simulink model "ballonplate_correctordinates29062016"  (R2016a)
settings: Solver=ode3  StartTime=0.0  StopTime=100  FixedStep=T  RelTol=1e-3
values from neighbouring files (symbols this model uses):
  T = 0.01    [paramters.m]
undefined symbols (not defined in the file or in its folder): initial_position, initial_velocity
libraries: vrlib x10, simulink x5, fuzblock x2
settings Model: Creator=akhan  LastModifiedBy=akhan
settings DataIOCC: LimitDataPoints=on  SaveFormat=Array
settings DebuggingCC: SolverPrmCheckMsg=warning
settings HardwareCC: ProdBitPerPointer=32  ProdLargestAtomicFloat=None  ProdIntDivRoundTo=Undefined  ProdEndianess=Unspecified  ProdWordSize=32  ProdHWDeviceType=32-bit Generic
settings ModelReferenceCC: PropagateSignalLabelsOutOfModel=off
settings ConfigComp: CovModelRefEnable=Off  CovSFcnEnable=off

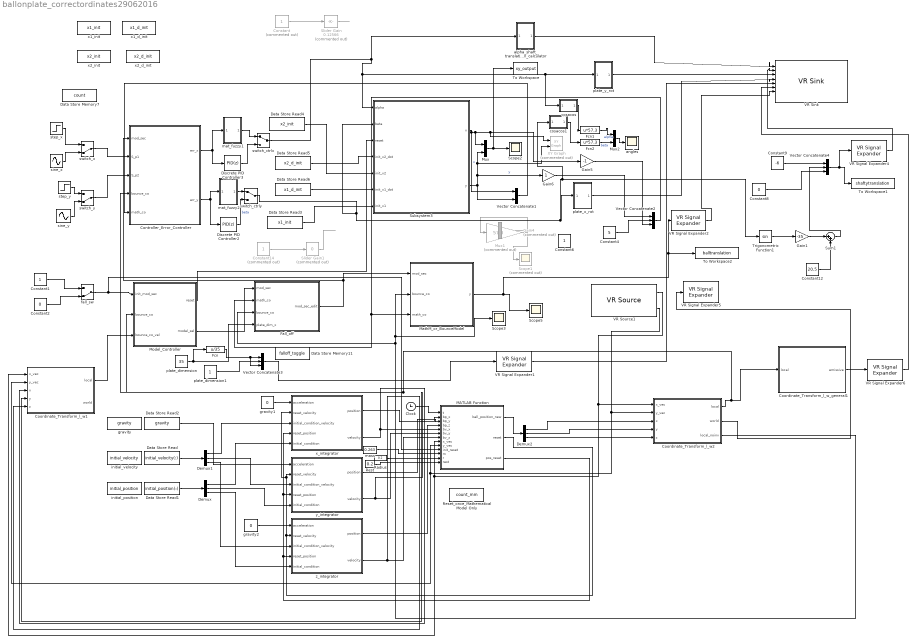
== system ballonplate_correctordinates29062016 ==
  Clock : Clock
  Constant : Constant  Commented=on
  Constant1 : Constant
  Constant12 : Constant  Value=20.5
  Constant14 : Constant  Commented=on
  Constant2 : Constant  Value=0
  Constant4 : Constant  Value=5
  Constant6 : Constant
  Constant8 : Constant  Value=0
  Constant9 : Constant  Value=-6
  Controller_Error_Controller : MATLAB Function  TreatAsAtomicUnit=on
  Coordinate_Transform_l_w1 : MATLAB Function  TreatAsAtomicUnit=on
  Coordinate_Transform_l_w2 : MATLAB Function  TreatAsAtomicUnit=on
  Coordinate_Transform_l_w_general1 : MATLAB Function  TreatAsAtomicUnit=on
  Data Store Memory11 : DataStoreMemory  DataStoreName=falloff_toggle  ShowAdditionalParam=off  OutDataTypeStr=double
  Data Store Memory7 : DataStoreMemory  DataStoreName=count  ShowAdditionalParam=off  OutDataTypeStr=double
  Data Store Read : DataStoreRead  DataStoreName=initial_velocity  DataStoreElements=initial_velocity(:)
  Data Store Read1 : DataStoreRead  DataStoreName=initial_position  DataStoreElements=initial_position(:)
  Data Store Read2 : DataStoreRead  DataStoreName=gravity  DataStoreElements=gravity
  Data Store Read3 : DataStoreRead  DataStoreName=x1_init  DataStoreElements=x1_init
  Data Store Read4 : DataStoreRead  DataStoreName=x2_init  DataStoreElements=x2_init
  Data Store Read5 : DataStoreRead  DataStoreName=x2_d_init  DataStoreElements=x2_d_init
  Data Store Read6 : DataStoreRead  DataStoreName=x1_d_init  DataStoreElements=x1_d_init
  Demux : Demux  Outputs=3
  Demux1 : Demux  Outputs=3
  Demux2 : Demux  Outputs=3
  Discrete PID Controller2 : simulink/Continuous/PID Controller  Controller=PID  TimeDomain=Discrete-time  SampleTime=T  IntegratorMethod=Backward Euler  FilterMethod=Forward Euler  Form=Parallel  UseFilter=on  ControllerParametersSource=internal  P=0.0496279719669994  I=0.00120600765535881  D=0.453206483387622  N=36.9012017074974  InitialConditionSource=internal  InitialConditionForIntegrator=0  InitialConditionForFilter=0  ExternalReset=none  LimitOutput=on  UpperSaturationLimit=1  LowerSaturationLimit=-1  LinearizeAsGain=off  AntiWindupMode=none  Kb=1  TrackingMode=off  Kt=1  PParamMin=[]  PParamMax=[]  IParamMin=[]  IParamMax=[]  DParamMin=[]  DParamMax=[]  NParamMin=[]  NParamMax=[]  KbParamMin=[]  KbParamMax=[]  KtParamMin=[]  KtParamMax=[]  POutMin=[]  POutMax=[]  IOutMin=[]  IOutMax=[]  DOutMin=[]  DOutMax=[]  NOutMin=[]  NOutMax=[]  KbOutMin=[]  KbOutMax=[]  KtOutMin=[]  KtOutMax=[]  IntegratorOutMin=[]  IntegratorOutMax=[]  FilterOutMin=[]  FilterOutMax=[]  SumOutMin=[]  SumOutMax=[]  SumI1OutMin=[]  SumI1OutMax=[]  SumI2OutMin=[]  SumI2OutMax=[]  SumI3OutMin=[]  SumI3OutMax=[]  SumDOutMin=[]  SumDOutMax=[]  SaturationOutMin=[]  SaturationOutMax=[]  IntegratorContinuousStateAttributes=''  IntegratorStateMustResolveToSignalObject=off  IntegratorRTWStateStorageClass=Auto  FilterContinuousStateAttributes=''  FilterStateMustResolveToSignalObject=off  FilterRTWStateStorageClass=Auto  DifferentiatorICPrevScaledInput=0  DifferentiatorOutMin=[]  DifferentiatorOutMax=[]
  Discrete PID Controller3 : simulink/Continuous/PID Controller  Controller=PID  TimeDomain=Discrete-time  SampleTime=T  IntegratorMethod=Backward Euler  FilterMethod=Forward Euler  Form=Parallel  UseFilter=on  ControllerParametersSource=internal  P=0.0496279719669994  I=0.00120600765535881  D=0.453206483387622  N=36.9012017074974  InitialConditionSource=internal  InitialConditionForIntegrator=0  InitialConditionForFilter=0  ExternalReset=none  LimitOutput=on  UpperSaturationLimit=1  LowerSaturationLimit=-1  LinearizeAsGain=off  AntiWindupMode=none  Kb=1  TrackingMode=off  Kt=1  PParamMin=[]  PParamMax=[]  IParamMin=[]  IParamMax=[]  DParamMin=[]  DParamMax=[]  NParamMin=[]  NParamMax=[]  KbParamMin=[]  KbParamMax=[]  KtParamMin=[]  KtParamMax=[]  POutMin=[]  POutMax=[]  IOutMin=[]  IOutMax=[]  DOutMin=[]  DOutMax=[]  NOutMin=[]  NOutMax=[]  KbOutMin=[]  KbOutMax=[]  KtOutMin=[]  KtOutMax=[]  IntegratorOutMin=[]  IntegratorOutMax=[]  FilterOutMin=[]  FilterOutMax=[]  SumOutMin=[]  SumOutMax=[]  SumI1OutMin=[]  SumI1OutMax=[]  SumI2OutMin=[]  SumI2OutMax=[]  SumI3OutMin=[]  SumI3OutMax=[]  SumDOutMin=[]  SumDOutMax=[]  SaturationOutMin=[]  SaturationOutMax=[]  IntegratorContinuousStateAttributes=''  IntegratorStateMustResolveToSignalObject=off  IntegratorRTWStateStorageClass=Auto  FilterContinuousStateAttributes=''  FilterStateMustResolveToSignalObject=off  FilterRTWStateStorageClass=Auto  DifferentiatorICPrevScaledInput=0  DifferentiatorOutMin=[]  DifferentiatorOutMax=[]
  Fall_off : MATLAB Function  TreatAsAtomicUnit=on
  Fcn : Fcn  Expr=u/35
  Fcn1 : Fcn  Expr=u*57.3
  Fcn2 : Fcn  Expr=u*57.3
  Gain1 : Gain  Gain=-35
  Gain4 : Gain  Commented=on  Gain=57.3  SampleTime=T
  Gain5 : Gain  Gain=-1
  Gain6 : Gain
  MATLAB Function : MATLAB Function  TreatAsAtomicUnit=on
  MathM_or_BounceModel : MATLAB Function  TreatAsAtomicUnit=on
  Model_Controller : MATLAB Function  TreatAsAtomicUnit=on
  Mux : Mux  Inputs=2
  Mux1 : Mux  Commented=on  Inputs=2
  Mux2 : Mux  Inputs=2
  Radius : Constant  Value=0.2
  Reset_once_Mathematical Model Only : DataStoreMemory  DataStoreName=count_mm  ShowAdditionalParam=off  OutDataTypeStr=double
  Rest : Constant  Value=0.2
  Scope1 : Scope  Commented=on
  Scope2 : Scope
  Scope3 : Scope
  Scope5 : Scope
  Slider Gain : simulink/Math Operations/Slider Gain  Commented=on  low=-1.5708  gain=0.12566  high=1.5708
  Slider Gain1 : simulink/Math Operations/Slider Gain  Commented=on  low=-1.5708  gain=0  high=1.57
  Subsystem3 : Subsystem  mask{m=0.263, r=0.2}
      mask prompts: m "Mass"; r "Radius"
      mask Display:
      | image('bp.jpg')
      | port_label('input',1,'alpha')
      | port_label('input',2,'beta')
      | port_label('input',3,'reset')
      | port_label('input',4,'x2_dot_init')
      | port_label('input',5,'x2_init')
      | port_label('input',6,'x1_dot_init')
      | port_label('input',7,'x1_init')
      | port_label('output',1,'x')
      | port_label('output',2,'y')
  Sum1 : Sum  Inputs=|++
  To Workspace : ToWorkspace  VariableName=xy_output  SaveFormat=Timeseries  SampleTime=T
  To Workspace1 : ToWorkspace  VariableName=shaftytranslation  SaveFormat=Timeseries  SampleTime=T
  To Workspace2 : ToWorkspace  VariableName=balltranslation  SaveFormat=Timeseries  SampleTime=T
  Trigonometric Function1 : Trigonometry
  VR Signal Expander{1,4..6} (4 alike) : vrlib/VR Signal Expander  outwidth=3  outidx=[1 2 3]
  VR Signal Expander2 : vrlib/VR Signal Expander  outwidth=3  outidx=[3 2 1]
  VR Sink : vrlib/VR Sink  InstantiateOnLoad=on  SampleTime=-1  ViewEnable=on  RemoteChange=off  RemoteView=off  FieldsWritten=shaft_x.translation.3.1.1.double#shaft_y.translation.3.1.1.double#plate_test_y.rotation.4.1.1.double#plate_test_x.rotation.4.1.1.double#plate_trans.scale.3.1.1.double#plate_mat.emissiveColor.3.1.1.double#ball_trans.translation.3.1.1.double#world_ball.translation.3.1.1.double  WorldFileName=bandplate_move_correctordinates.wrl  AutoView=off  VideoDimensions=[]  AllowVariableSize=off
  VR Source1 : vrlib/VR Source  InstantiateOnLoad=on  SampleTime=-1  ViewEnable=on  RemoteChange=off  RemoteView=off  FieldsRead=reference_x.translation_abs.1.3.1.double#reference_y.translation_abs.1.3.1.double  WorldFileName=bandplate_move_correctordinates.wrl  AutoView=off  VideoDimensions=[]  AllowVariableSize=off
  Vector Concatenate1 : Concatenate
  Vector Concatenate2 : Concatenate  NumInputs=3
  Vector Concatenate3 : Concatenate  NumInputs=3
  Vector Concatenate4 : Concatenate  NumInputs=3
  XY Graph : simulink/Sinks/XY Graph  Commented=on  xmin=-35  xmax=35  ymin=-35  ymax=35  st=-1
  alpha_shaft_translation_calculator : Subsystem
  angles : Scope
  cosacos : Subsystem
  cosacos1 : Subsystem
  fall_sw : ManualSwitch  CurrentSetting=0
  gravity : DataStoreMemory  DataStoreName=gravity  InitialValue=-4  ShowAdditionalParam=off  OutDataTypeStr=double
  gravity1 : Constant  Value=0
  gravity2 : Constant  Value=0
  initial_position : DataStoreMemory  DataStoreName=initial_position  InitialValue=[5;25;3]  ShowAdditionalParam=off  OutDataTypeStr=double
  initial_velocity : DataStoreMemory  DataStoreName=initial_velocity  InitialValue=[0;5;0]  ShowAdditionalParam=off  OutDataTypeStr=double
  mass : Constant  Value=0.263
  mat_fuzzy1 : Subsystem
  mat_fuzzy2 : Subsystem
  plate_dimension : Constant  Value=35
  plate_dimension1 : Constant
  plate_x_rot : Subsystem
  plate_y_rot : Subsystem
  sine_x : Sin  Amplitude=5  Frequency=0.1  SampleTime=0
  sine_y : Sin  Amplitude=5  Frequency=0.1  Phase=-pi/2  SampleTime=0
  step_x : Step  Time=0  After=5  SampleTime=0
  step_y : Step  Time=0  After=5  SampleTime=0
  switch_ctrlx : ManualSwitch
  switch_ctrly : ManualSwitch
  switch_x : ManualSwitch  CurrentSetting=0
  switch_y : ManualSwitch  CurrentSetting=0
  x1_d_init : DataStoreMemory  DataStoreName=x1_d_init  ShowAdditionalParam=off  OutDataTypeStr=double
  x1_init : DataStoreMemory  DataStoreName=x1_init  ShowAdditionalParam=off  OutDataTypeStr=double
  x2_d_init : DataStoreMemory  DataStoreName=x2_d_init  ShowAdditionalParam=off  OutDataTypeStr=double
  x2_init : DataStoreMemory  DataStoreName=x2_init  ShowAdditionalParam=off  OutDataTypeStr=double
  x_integrator : Subsystem
  y_integrator : Subsystem
  z_integrator : Subsystem
  wires:
  Subsystem3/1(x) -> Vector Concatenate1/1, XY Graph/1, Gain5/1, Mux/1  "x"
  Subsystem3/2(y) -> XY Graph/2, Mux/2, Gain6/1, Vector Concatenate1/2  "y"
  Mux1/1 -> Gain4/1
  Gain4/1 -> Scope1/1
  Constant4/1 -> Vector Concatenate2/2
  Vector Concatenate2/1 -> Fall_off/2(math_co), MathM_or_BounceModel/3(math_co)
  Vector Concatenate4/1 -> To Workspace1/1, VR Signal Expander4/1
  Constant9/1 -> Vector Concatenate4/1
  Constant8/1 -> Vector Concatenate4/3
  Trigonometric Function1/1 -> Gain1/1
  Gain1/1 -> Sum1/1
  Constant12/1 -> Sum1/2
  Sum1/1 -> Vector Concatenate4/2
  Gain5/1 -> Vector Concatenate2/3
  Gain6/1 -> Vector Concatenate2/1
  Constant/1 -> Slider Gain/1
  Constant14/1 -> Slider Gain1/1
  Slider Gain/1 -> ?
  switch_ctrlx/1 -> Subsystem3/1(alpha), cosacos/1(In1), plate_y_rot/1(In1), alpha_shaft_translation_calculator/1(In1)
  Slider Gain1/1 -> ?
  switch_ctrly/1 -> cosacos1/1(In1), Trigonometric Function1/1, plate_x_rot/1(In1), Subsystem3/2(beta)
  VR Source1/1 -> Coordinate_Transform_l_w2/1(x_vec), MATLAB Function/8(x_vec), Coordinate_Transform_l_w1/1(x_vec)
  VR Source1/2 -> Coordinate_Transform_l_w2/2(y_vec), MATLAB Function/9(y_vec), Coordinate_Transform_l_w1/2(y_vec)
  Coordinate_Transform_l_w2/2(world) -> VR Signal Expander5/1
  Coordinate_Transform_l_w2/1(local) -> Controller_Error_Controller/4(bounce_co), Model_Controller/2(bounce_co), Coordinate_Transform_l_w_general1/1(local)
  Coordinate_Transform_l_w_general1/1(emissive) -> VR Signal Expander6/1
  Data Store Read2/1 -> y_integrator/1(acceleration)
  x_integrator/1(position) -> MATLAB Function/2(bp_x)
  y_integrator/1(position) -> MATLAB Function/3(bp_y)
  z_integrator/1(position) -> MATLAB Function/4(bp_z)
  x_integrator/2(velocity) -> Coordinate_Transform_l_w1/3(x), MATLAB Function/5(bv_x)
  y_integrator/2(velocity) -> Coordinate_Transform_l_w1/4(y), MATLAB Function/6(bv_y)
  z_integrator/2(velocity) -> Coordinate_Transform_l_w1/5(z), MATLAB Function/7(bv_z)
  Demux/1 -> x_integrator/5(initial_condition)
  Demux/2 -> y_integrator/5(initial_condition)
  Demux/3 -> z_integrator/5(initial_condition)
  Demux1/1 -> x_integrator/3(initial_condition_velocity)
  Demux1/2 -> y_integrator/3(initial_condition_velocity)
  Demux1/3 -> z_integrator/3(initial_condition_velocity)
  gravity1/1 -> x_integrator/1(acceleration)
  gravity2/1 -> z_integrator/1(acceleration)
  MATLAB Function/1(ball_position_new) -> Demux2/1
  Demux2/1 -> Coordinate_Transform_l_w2/3(x)
  Demux2/2 -> Coordinate_Transform_l_w2/4(y)
  Demux2/3 -> Coordinate_Transform_l_w2/5(z)
  MATLAB Function/2(reset) -> z_integrator/2(reset_velocity), x_integrator/2(reset_velocity), y_integrator/2(reset_velocity)
  Data Store Read/1 -> Demux1/1
  Data Store Read1/1 -> Demux/1
  MATLAB Function/3(pos_reset) -> x_integrator/4(reset_position), y_integrator/4(reset_position), z_integrator/4(reset_position)
  Clock/1 -> MATLAB Function/1(t)
  Mux/1 -> To Workspace/1, Scope2/1
  Data Store Read5/1 -> Subsystem3/4(init_x2_dot)
  Data Store Read6/1 -> Subsystem3/6(init_x1_dot)
  Data Store Read4/1 -> Subsystem3/5(init_x2)
  Data Store Read3/1 -> Subsystem3/7(init_x1)
  Model_Controller/1(reset) -> Subsystem3/3(reset)
  Coordinate_Transform_l_w2/3(local_noinv) -> Fall_off/3(bounce_co), MathM_or_BounceModel/2(bounce_co), Scope3/1
  fall_sw/1 -> MATLAB Function/10(init_reset), Model_Controller/1(init_mod_sec)
  Constant1/1 -> fall_sw/1
  Constant2/1 -> fall_sw/2
  Vector Concatenate1/1 -> Controller_Error_Controller/5(math_co)
  Coordinate_Transform_l_w1/1(local) -> Model_Controller/3(bounce_co_vel)
  Model_Controller/2(model_sel) -> Fall_off/1(mod_sec)
  Fall_off/1(mod_sec_edit) -> Controller_Error_Controller/1(mod_sec), MathM_or_BounceModel/1(mod_sec)
  MathM_or_BounceModel/1(y) -> To Workspace2/1, VR Signal Expander2/1, Scope5/1
  step_y/1 -> switch_y/1
  sine_y/1 -> switch_y/2
  switch_y/1 -> Controller_Error_Controller/3(S_p2)
  switch_x/1 -> Controller_Error_Controller/2(S_p1)
  sine_x/1 -> switch_x/2
  plate_dimension/1 -> Fcn/1, Fall_off/4(plate_dim_x)
  alpha_shaft_translation_calculator/1(Out1) -> VR Sink/1
  VR Signal Expander4/1 -> VR Sink/2
  plate_y_rot/1(Out1) -> VR Sink/3
  plate_x_rot/1(Out1) -> VR Sink/4
  VR Signal Expander6/1 -> VR Sink/6
  VR Signal Expander2/1 -> VR Sink/7
  Fcn/1 -> Vector Concatenate3/3, Vector Concatenate3/1
  plate_dimension1/1 -> Vector Concatenate3/2
  Vector Concatenate3/1 -> VR Signal Expander1/1
  VR Signal Expander1/1 -> VR Sink/5
  Rest/1 -> MATLAB Function/13(rest)
  mass/1 -> MATLAB Function/11(m)
  Radius/1 -> MATLAB Function/12(r)
  Fcn1/1 -> Mux2/1  "alpha"
  Fcn2/1 -> Mux2/2  "beta"
  Mux2/1 -> angles/1
  cosacos/1(Out1) -> Fcn1/1
  cosacos1/1(Out1) -> Fcn2/1
  Controller_Error_Controller/2(err_y) -> Discrete PID Controller2/1, mat_fuzzy2/1(In1)
  step_x/1 -> switch_x/1
  mat_fuzzy1/1(Out1) -> switch_ctrlx/1
  Discrete PID Controller3/1 -> switch_ctrlx/2
  Controller_Error_Controller/1(err_x) -> Discrete PID Controller3/1, mat_fuzzy1/1(In1)
  mat_fuzzy2/1(Out1) -> switch_ctrly/1
  Discrete PID Controller2/1 -> switch_ctrly/2  "beta"

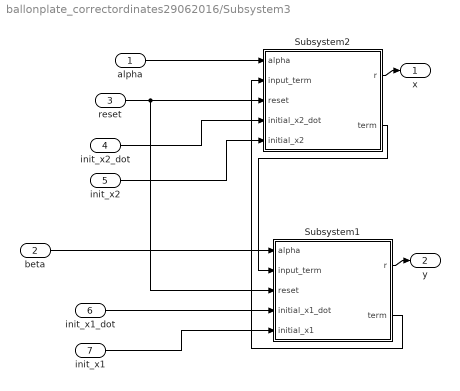
== system ballonplate_correctordinates29062016/Subsystem3 ==
  alpha : Inport
  beta : Inport  Port=2
  reset : Inport  Port=3
  init_x2_dot : Inport  Port=4
  init_x2 : Inport  Port=5
  init_x1_dot : Inport  Port=6
  init_x1 : Inport  Port=7
  Subsystem1 : Subsystem
  Subsystem2 : Subsystem
  x : Outport
  y : Outport  Port=2
  wires:
  Subsystem1/2(term) -> Subsystem2/2(input_term)
  beta/1 -> Subsystem1/1(alpha)
  alpha/1 -> Subsystem2/1(alpha)
  Subsystem1/1(r) -> y/1
  Subsystem2/1(r) -> x/1
  Subsystem2/2(term) -> Subsystem1/2(input_term)
  reset/1 -> Subsystem1/3(reset), Subsystem2/3(reset)
  init_x2_dot/1 -> Subsystem2/4(initial_x2_dot)
  init_x2/1 -> Subsystem2/5(initial_x2)
  init_x1_dot/1 -> Subsystem1/4(initial_x1_dot)
  init_x1/1 -> Subsystem1/5(initial_x1)

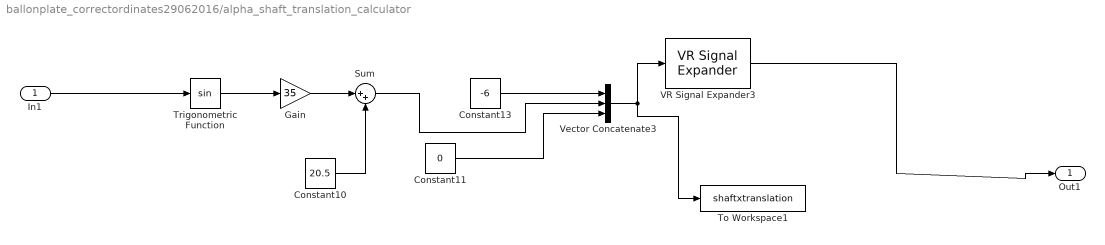
== system ballonplate_correctordinates29062016/alpha_shaft_translation_calculator ==
  In1 : Inport
  Constant10 : Constant  Value=20.5
  Constant11 : Constant  Value=0
  Constant13 : Constant  Value=-6
  Gain : Gain  Gain=35
  Sum : Sum  Inputs=|++
  To Workspace1 : ToWorkspace  VariableName=shaftxtranslation  SaveFormat=Timeseries  SampleTime=T
  Trigonometric Function : Trigonometry
  VR Signal Expander3 : vrlib/VR Signal Expander  outwidth=3  outidx=[1 2 3]
  Vector Concatenate3 : Concatenate  NumInputs=3
  Out1 : Outport
  wires:
  Constant11/1 -> Vector Concatenate3/3
  Vector Concatenate3/1 -> VR Signal Expander3/1, To Workspace1/1
  Constant13/1 -> Vector Concatenate3/1
  Gain/1 -> Sum/1
  Constant10/1 -> Sum/2
  Trigonometric Function/1 -> Gain/1
  Sum/1 -> Vector Concatenate3/2
  VR Signal Expander3/1 -> Out1/1
  In1/1 -> Trigonometric Function/1

== system ballonplate_correctordinates29062016/cosacos ==
  In1 : Inport
  Trigonometric Function3 : Trigonometry  Operator=acos
  Trigonometric Function4 : Trigonometry  Operator=cos
  Out1 : Outport
  wires:
  In1/1 -> Trigonometric Function4/1
  Trigonometric Function3/1 -> Out1/1
  Trigonometric Function4/1 -> Trigonometric Function3/1

== system ballonplate_correctordinates29062016/cosacos1 ==
  In1 : Inport
  Trigonometric Function3 : Trigonometry  Operator=acos
  Trigonometric Function4 : Trigonometry  Operator=cos
  Out1 : Outport
  wires:
  In1/1 -> Trigonometric Function4/1
  Trigonometric Function3/1 -> Out1/1
  Trigonometric Function4/1 -> Trigonometric Function3/1

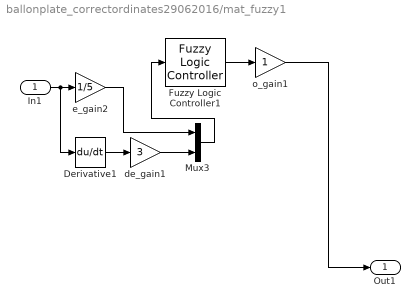
== system ballonplate_correctordinates29062016/mat_fuzzy1 ==
  In1 : Inport
  Derivative1 : Derivative
  Fuzzy Logic Controller1 : fuzblock/Fuzzy Logic  Controller  fis='ball_plate_normalized.fis'
  Mux3 : Mux  Inputs=2
  de_gain1 : Gain  Gain=3
  e_gain2 : Gain  Gain=1/5
  o_gain1 : Gain
  Out1 : Outport
  wires:
  e_gain2/1 -> Mux3/1
  Mux3/1 -> Fuzzy Logic Controller1/1
  Fuzzy Logic Controller1/1 -> o_gain1/1
  de_gain1/1 -> Mux3/2
  Derivative1/1 -> de_gain1/1
  In1/1 -> Derivative1/1, e_gain2/1
  o_gain1/1 -> Out1/1

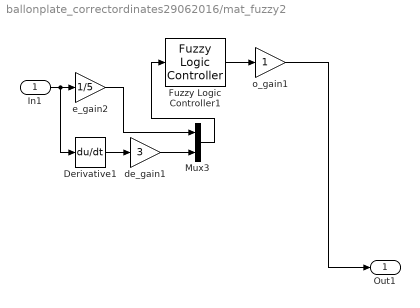
== system ballonplate_correctordinates29062016/mat_fuzzy2 ==
  In1 : Inport
  Derivative1 : Derivative
  Fuzzy Logic Controller1 : fuzblock/Fuzzy Logic  Controller  fis='ball_plate_normalized.fis'
  Mux3 : Mux  Inputs=2
  de_gain1 : Gain  Gain=3
  e_gain2 : Gain  Gain=1/5
  o_gain1 : Gain
  Out1 : Outport
  wires:
  e_gain2/1 -> Mux3/1
  Mux3/1 -> Fuzzy Logic Controller1/1
  Fuzzy Logic Controller1/1 -> o_gain1/1
  de_gain1/1 -> Mux3/2
  Derivative1/1 -> de_gain1/1
  In1/1 -> Derivative1/1, e_gain2/1
  o_gain1/1 -> Out1/1

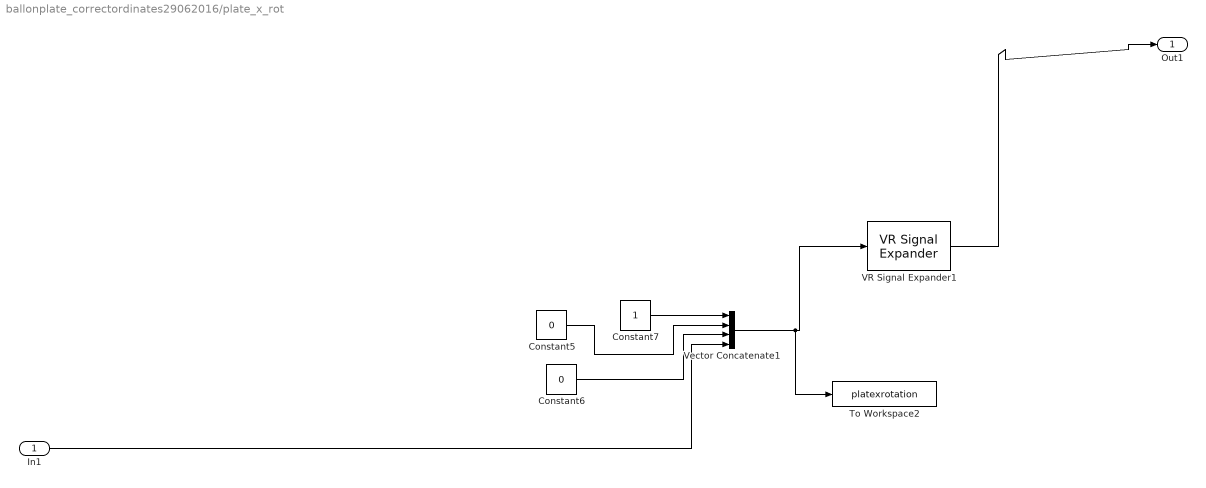
== system ballonplate_correctordinates29062016/plate_x_rot ==
  In1 : Inport
  Constant5 : Constant  Value=0
  Constant6 : Constant  Value=0
  Constant7 : Constant
  To Workspace2 : ToWorkspace  VariableName=platexrotation  SaveFormat=Timeseries  SampleTime=T
  VR Signal Expander1 : vrlib/VR Signal Expander  outwidth=4  outidx=[1 2 3 4]
  Vector Concatenate1 : Concatenate  NumInputs=4
  Out1 : Outport
  wires:
  Constant6/1 -> Vector Concatenate1/3
  Constant5/1 -> Vector Concatenate1/2
  Vector Concatenate1/1 -> To Workspace2/1, VR Signal Expander1/1
  Constant7/1 -> Vector Concatenate1/1
  VR Signal Expander1/1 -> Out1/1
  In1/1 -> Vector Concatenate1/4

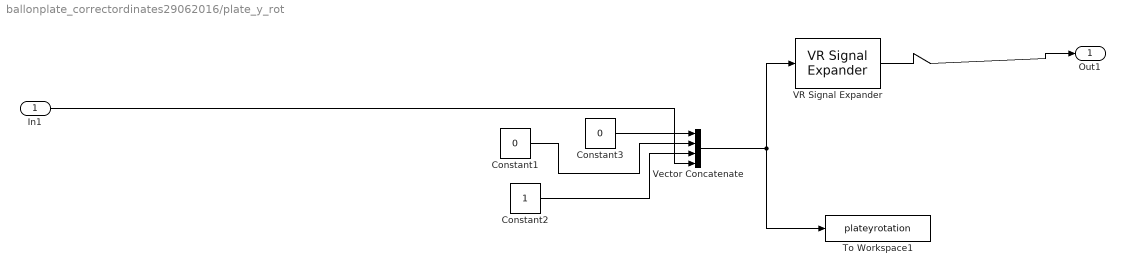
== system ballonplate_correctordinates29062016/plate_y_rot ==
  In1 : Inport
  Constant1 : Constant  Value=0
  Constant2 : Constant
  Constant3 : Constant  Value=0
  To Workspace1 : ToWorkspace  VariableName=plateyrotation  SaveFormat=Timeseries  SampleTime=-1
  VR Signal Expander : vrlib/VR Signal Expander  outwidth=4  outidx=[1 2 3 4]
  Vector Concatenate : Concatenate  NumInputs=4
  Out1 : Outport
  wires:
  Vector Concatenate/1 -> To Workspace1/1, VR Signal Expander/1
  Constant2/1 -> Vector Concatenate/3
  Constant1/1 -> Vector Concatenate/2
  Constant3/1 -> Vector Concatenate/1
  VR Signal Expander/1 -> Out1/1
  In1/1 -> Vector Concatenate/4

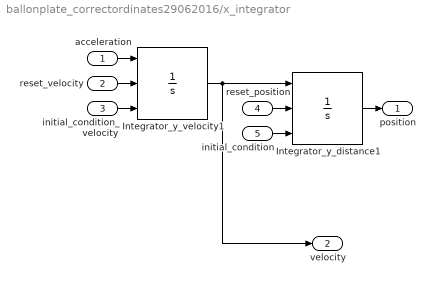
== system ballonplate_correctordinates29062016/x_integrator ==
  acceleration : Inport
  reset_velocity : Inport  Port=2
  initial_condition_velocity : Inport  Port=3
  reset_position : Inport  Port=4
  initial_condition : Inport  Port=5
  Integrator_y_distance1 : Integrator  ExternalReset=rising  InitialConditionSource=external
  Integrator_y_velocity1 : Integrator  ExternalReset=rising  InitialConditionSource=external
  position : Outport
  velocity : Outport  Port=2
  wires:
  Integrator_y_velocity1/1 -> velocity/1, Integrator_y_distance1/1
  reset_position/1 -> Integrator_y_distance1/2
  Integrator_y_distance1/1 -> position/1
  initial_condition_velocity/1 -> Integrator_y_velocity1/3
  initial_condition/1 -> Integrator_y_distance1/3
  reset_velocity/1 -> Integrator_y_velocity1/2
  acceleration/1 -> Integrator_y_velocity1/1

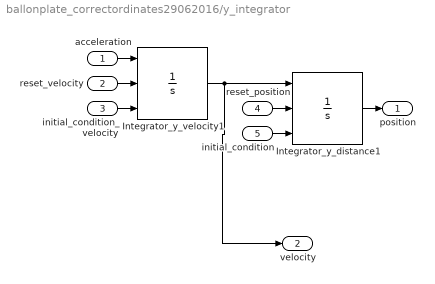
== system ballonplate_correctordinates29062016/y_integrator ==
  acceleration : Inport
  reset_velocity : Inport  Port=2
  initial_condition_velocity : Inport  Port=3
  reset_position : Inport  Port=4
  initial_condition : Inport  Port=5
  Integrator_y_distance1 : Integrator  ExternalReset=rising  InitialConditionSource=external
  Integrator_y_velocity1 : Integrator  ExternalReset=rising  InitialConditionSource=external
  position : Outport
  velocity : Outport  Port=2
  wires:
  Integrator_y_velocity1/1 -> velocity/1, Integrator_y_distance1/1
  reset_position/1 -> Integrator_y_distance1/2
  Integrator_y_distance1/1 -> position/1
  initial_condition_velocity/1 -> Integrator_y_velocity1/3
  initial_condition/1 -> Integrator_y_distance1/3
  reset_velocity/1 -> Integrator_y_velocity1/2
  acceleration/1 -> Integrator_y_velocity1/1

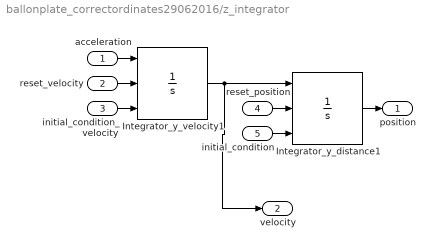
== system ballonplate_correctordinates29062016/z_integrator ==
  acceleration : Inport
  reset_velocity : Inport  Port=2
  initial_condition_velocity : Inport  Port=3
  reset_position : Inport  Port=4
  initial_condition : Inport  Port=5
  Integrator_y_distance1 : Integrator  ExternalReset=rising  InitialConditionSource=external
  Integrator_y_velocity1 : Integrator  ExternalReset=rising  InitialConditionSource=external
  position : Outport
  velocity : Outport  Port=2
  wires:
  Integrator_y_velocity1/1 -> velocity/1, Integrator_y_distance1/1
  reset_position/1 -> Integrator_y_distance1/2
  Integrator_y_distance1/1 -> position/1
  initial_condition_velocity/1 -> Integrator_y_velocity1/3
  initial_condition/1 -> Integrator_y_distance1/3
  reset_velocity/1 -> Integrator_y_velocity1/2
  acceleration/1 -> Integrator_y_velocity1/1

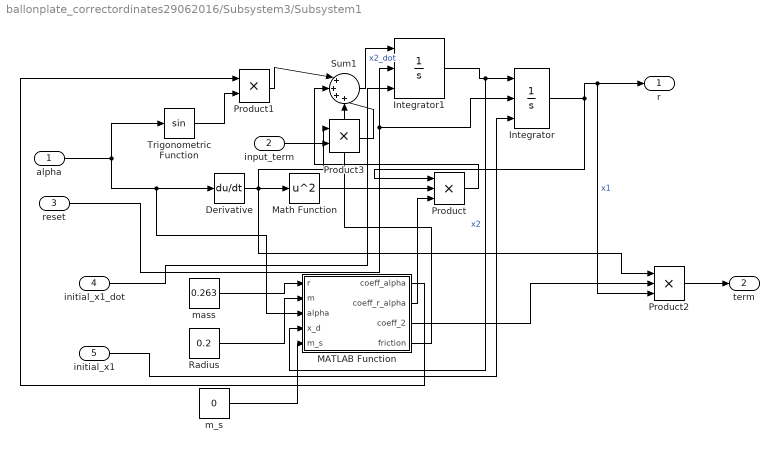
== system ballonplate_correctordinates29062016/Subsystem3/Subsystem1 ==
  alpha : Inport
  input_term : Inport  Port=2
  reset : Inport  Port=3
  initial_x1_dot : Inport  Port=4
  initial_x1 : Inport  Port=5
  Derivative : Derivative
  Integrator : Integrator  ExternalReset=rising  InitialConditionSource=external  InitialCondition=0.004427
  Integrator1 : Integrator  ExternalReset=rising  InitialConditionSource=external
  MATLAB Function : MATLAB Function  TreatAsAtomicUnit=on
  Math Function : Math  Operator=square  SaturateOnIntegerOverflow=on
  Product : Product  Inputs=3
  Product1 : Product
  Product2 : Product  Inputs=3
  Product3 : Product
  Radius : Constant  Value=0.2
  Sum1 : Sum  Inputs=|++++
  Trigonometric Function : Trigonometry
  m_s : Constant  Value=0
  mass : Constant  Value=0.263
  r : Outport
  term : Outport  Port=2
  wires:
  Product1/1 -> Sum1/1
  Derivative/1 -> Product2/1, Product3/1, Math Function/1
  Sum1/1 -> Integrator1/1  "x2_dot"
  Integrator/1 -> Product2/3, r/1, Product/1  "x1"
  Product/1 -> Sum1/2
  Integrator1/1 -> MATLAB Function/4(x_d), Integrator/1  "x2"
  Trigonometric Function/1 -> Product1/2
  alpha/1 -> MATLAB Function/3(alpha), Derivative/1, Trigonometric Function/1
  Math Function/1 -> Product/2
  mass/1 -> MATLAB Function/1(r)
  Radius/1 -> MATLAB Function/2(m)
  MATLAB Function/1(coeff_alpha) -> Product1/1
  MATLAB Function/2(coeff_r_alpha) -> Product/3
  MATLAB Function/3(coeff_2) -> Product2/2
  Product2/1 -> term/1
  input_term/1 -> Product3/2
  Product3/1 -> Sum1/3
  reset/1 -> Integrator/2, Integrator1/2
  initial_x1_dot/1 -> Integrator1/3
  initial_x1/1 -> Integrator/3
  MATLAB Function/4(friction) -> Sum1/4
  m_s/1 -> MATLAB Function/5(m_s)

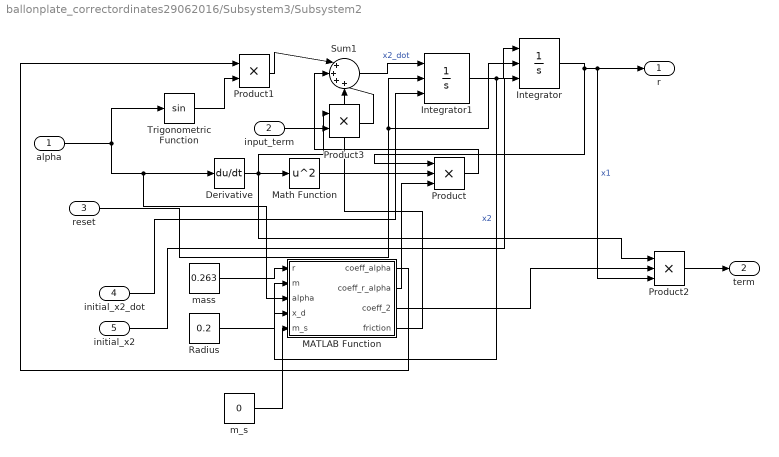
== system ballonplate_correctordinates29062016/Subsystem3/Subsystem2 ==
  alpha : Inport
  input_term : Inport  Port=2
  reset : Inport  Port=3
  initial_x2_dot : Inport  Port=4
  initial_x2 : Inport  Port=5
  Derivative : Derivative
  Integrator : Integrator  ExternalReset=rising  InitialConditionSource=external  InitialCondition=0.004427
  Integrator1 : Integrator  ExternalReset=rising  InitialConditionSource=external
  MATLAB Function : MATLAB Function  TreatAsAtomicUnit=on
  Math Function : Math  Operator=square  SaturateOnIntegerOverflow=on
  Product : Product  Inputs=3
  Product1 : Product
  Product2 : Product  Inputs=3
  Product3 : Product
  Radius : Constant  Value=0.2
  Sum1 : Sum  Inputs=|++++
  Trigonometric Function : Trigonometry
  m_s : Constant  Value=0
  mass : Constant  Value=0.263
  r : Outport
  term : Outport  Port=2
  wires:
  Product1/1 -> Sum1/1
  Derivative/1 -> Product2/1, Product3/1, Math Function/1
  Sum1/1 -> Integrator1/1  "x2_dot"
  Integrator/1 -> Product/1, Product2/3, r/1  "x1"
  Product/1 -> Sum1/2
  Integrator1/1 -> MATLAB Function/4(x_d), Integrator/1  "x2"
  Trigonometric Function/1 -> Product1/2
  alpha/1 -> MATLAB Function/3(alpha), Derivative/1, Trigonometric Function/1
  Math Function/1 -> Product/2
  mass/1 -> MATLAB Function/1(r)
  Radius/1 -> MATLAB Function/2(m)
  MATLAB Function/1(coeff_alpha) -> Product1/1
  MATLAB Function/2(coeff_r_alpha) -> Product/3
  MATLAB Function/3(coeff_2) -> Product2/2
  Product2/1 -> term/1
  input_term/1 -> Product3/2
  Product3/1 -> Sum1/3
  reset/1 -> Integrator/2, Integrator1/2
  initial_x2_dot/1 -> Integrator1/3
  initial_x2/1 -> Integrator/3
  MATLAB Function/4(friction) -> Sum1/4
  m_s/1 -> MATLAB Function/5(m_s)

== matlab function ballonplate_correctordinates29062016/Subsystem3/Subsystem1/MATLAB Function ==
  data: r input; coeff_alpha output; m input; coeff_r_alpha output; coeff_2 output; alpha input; x_d input; friction output; m_s input
function [coeff_alpha, coeff_r_alpha,coeff_2,friction] = fcn(r,m,alpha,x_d,m_s)
%#codeg
J=2*m*r*r/5;
coeff_r_alpha=m/((J/r*r)+m);
coeff_alpha=   -m*(-9.8)/((J/r*r)+m);
coeff_2=m/((J/r*r)+m);


m_s = 0;
friction = -m_s*m*9.8*cos(alpha)*sign(x_d);
friction = friction/((J/r*r)+m);

== matlab function ballonplate_correctordinates29062016/Subsystem3/Subsystem2/MATLAB Function ==
  data: r input; coeff_alpha output; m input; coeff_r_alpha output; coeff_2 output; alpha input; friction output; x_d input; m_s input
function [coeff_alpha, coeff_r_alpha,coeff_2,friction] = fcn(r,m,alpha,x_d,m_s)
%#codeg
J=2*m*r*r/5;
coeff_r_alpha=m/((J/r*r)+m);
coeff_alpha=   -m*(-9.8)/((J/r*r)+m);
coeff_2=m/((J/r*r)+m);


%coefficient of friction

friction = -m_s*m*9.8*cos(alpha)*sign(x_d);
friction = friction/((J/r*r)+m);

== matlab function ballonplate_correctordinates29062016/MathM_or_BounceModel ==
  data: mod_sec input; y output size=3; gravity data_store_memory; bounce_co input size=3; math_co input size=3
function y = fcn(mod_sec,bounce_co,math_co)
%mod_sec if 0 output is bounce_co
%if anything else math_co
%this requires bounce_co and math_co for vrml model, note doesn't require
%the negative
if mod_sec == 1
    y = bounce_co;
elseif mod_sec == 0
    y = math_co;
else
    y = [2000 2000 2000]';
end

== matlab function ballonplate_correctordinates29062016/Controller_Error_Controller ==
  data: mod_sec input; S_p1 input; S_p2 input; err_x output; gravity data_store_memory; bounce_co input; math_co input size=2; err_y output
function [err_x,err_y] = fcn(mod_sec,S_p1,S_p2,bounce_co,math_co)
%this function requires the bounce_co and math_co for the mathematical
%model coordinates
threshold_for_touch = 3;
if mod_sec == 3
err_x = 0;
err_y = 0;
else
    if mod_sec == 0
        err_x = S_p1 - math_co(1);
        err_y = S_p2 - math_co(2);
    %threshold for touch
    elseif bounce_co(3)<= threshold_for_touch
        err_x = S_p1 - bounce_co(1);
        err_y = S_p2 - bounce_co(2);
    else err_x = 0;
         err_y = 0;
    end
end

== matlab function ballonplate_correctordinates29062016/Model_Controller ==
  data: init_mod_sec input; reset output; gravity data_store_memory; bounce_co input; bounce_co_vel input; model_sel output; x1_init data_store_memory; x1_d_init data_store_memory; x2_init data_store_memory; x2_d_init data_store_memory; initial_velocity data_store_memory; initial_position data_store_memory; count data_store_memory
function [reset,model_sel] = fcn(init_mod_sec,bounce_co,bounce_co_vel)
%mod_sec if 0 output is math_co
%if anything else math_co
%this requires the bounce_co in mathematical model coordinates
%probably need a count variable to stop resetting x1_init
global gravity;
global x1_init;
global x1_d_init;
global x2_init;
global x2_d_init;
global initial_velocity;
global initial_position;
global count;



    if init_mod_sec == 0
        gravity = 0;
        model_sel = 0;
        reset = 0;
        initial_position = [0;15;0];
        initial_velocity = [0;0;0];
    else 
        if gravity == 0
            if count <5
                reset = 1;
                x1_init = bounce_co(1);
                x2_init = bounce_co(2);
                x1_d_init = bounce_co_vel(1);
                x2_d_init = bounce_co_vel(2);
                count = count+1;
            else reset =1;
            end
        model_sel = 0;
        
        else reset = 0;
            model_sel = 1;
        end
    end

== matlab function ballonplate_correctordinates29062016/Coordinate_Transform_l_w2 ==
  data: x_vec input; y_vec input; x input; y input; local output; z input; world output; local_noinv output size=[1 3]
function [local,world,local_noinv] = fcn(x_vec,y_vec,x,y,z)
%y_p is y prime which is vector of y coordinate axis after rotation beta
%about the x axis
%x_p is rotation alpha about arbitary axis y_p
%This transformation gives the coordinates in the mathematical model
%coordinates
%x_vec -1 0 0
%y_vec 0 0 1
%z_vec 0 1 0
% This gives local where x is -x therefore x is correct and z 
%just need to swap x and z
world = [x;y;z];
z_vec=cross(x_vec,y_vec);
local=[x_vec,y_vec,z_vec]\[x;y;z];

%this gives local coordinates in vrml frame
local_noinv = [-local(1),local(3),local(2)];

%this gives local coordinates in ball and plate frame
temp = local(1);
local(1) = local(2);
local(2) = temp;

== matlab function ballonplate_correctordinates29062016/Coordinate_Transform_l_w_general1 ==
  data: local input; emissive output
function emissive = fcn(local)

if local(3)<5&(abs(local(2)))<35&(abs(local(3)))<35
    emissive = [0.8 0 0.2];
else emissive = [0 0 0.8];
end

== matlab function ballonplate_correctordinates29062016/MATLAB Function ==
  data: t input; bp_x input; ball_position_new output; bp_y input; bp_z input; bv_x input; bv_y input; bv_z input; reset output; initial_velocity data_store_memory; initial_position data_store_memory; gravity data_store_memory; x_vec input; y_vec input; pos_reset output; count_mm data_store_memory; init_reset input; m input; r input; rest input
function [ball_position_new,reset,pos_reset] = fcn(t,bp_x,bp_y,bp_z,bv_x,bv_y,bv_z,x_vec,y_vec,init_reset,m,r,rest)
%#codegen
global initial_velocity;
global initial_position;
global gravity;
global count_mm;

[local_pos,~]=coordinate_transform(x_vec,y_vec,bp_x,bp_y,bp_z);
ball_position=local_pos;
[local_vel,~]=coordinate_transform(x_vec,y_vec,bv_x,bv_y,bv_z);
ball_velocity=local_vel;
ball_position_new = [bp_x;bp_y;bp_z];
if (ball_position(3)<=3)&&t>0&&gravity~=0&&init_reset~=0
  reset=1;
 pos_reset=0;
% m = 0.263;
% r = 2;
J_sphere =0.4* m*r*r*eye(3);
J_sphere_inv = 2.5*eye(3)/(m*r*r);
% rest = 0.2;
ball_momentum = m*ball_velocity;
%This can change to reflect the plate
m_ground_inv = 0;
J_ground_inv = 0;
N = [0 0 1]';
%ball_position is ball centre which is all centre of gravity
contact_Point = [ball_position(1),ball_position(2),ball_position(3)-r]';
r_ball = contact_Point - ball_position;
%r_ground = contact_Point - ground_position;

kA = cross(r_ball,N);
%kB = cross(r_ground,N);
kB = [0 0 0];
uA = J_sphere_inv*kA;
uB = [0,0,0];
%ball_velocity - velocity of object B but ground is stationary
numer = -(1+rest)*(dot(N,ball_velocity));
denom = (1/m)+ m_ground_inv+dot(kA,uA);

f=numer/denom;
impulse = f*N;

ball_momentum = ball_momentum+impulse;
initial_velocity_temp = ball_momentum*1/m;
%parabolic extrapolation
a_para = 0.5*gravity;
b_para = initial_velocity_temp(3);
initial_velocity_temp = coordinate_transform_l_w(x_vec,y_vec,initial_velocity_temp(1),initial_velocity_temp(2),initial_velocity_temp(3));


turning_time = -b_para/(2*a_para);
%tolerance for resting contact
toler = 0.06;
if t~=0
if turning_time>=0
    turning_point = (a_para*turning_time*turning_time)+(b_para*turning_time);
    if turning_point<toler;
        initial_velocity = [0;0;0];
        %initial_position(2)=37.99;
        ball_position(2)=3;
        ball_position = coordinate_transform_l_w(x_vec,y_vec,ball_position(1),ball_position(2),ball_position(3));
        initial_position = ball_position;
        gravity = 0;
%testing position reset
        pos_reset=1;  
    else initial_velocity = initial_velocity_temp;
        pos_reset=0;
    end
else pos_reset=0;
end
end
% if t~=0
% plate_thickness = 1;
% interpenetration_index = plate_thickness + r;
% interpenetration_index = interpenetration_index - 0.25;
%     if local_pos(2)<= interpenetration_index
%         pos_reset = 1;
%         initial_velocity = [0;0;0];
%         initial_position(2)= plate_thickness + r;
%         gravity = 0;
%     else initial_velocity = initial_velocity_temp;
%     end
% end
else reset=0;
     pos_reset=0;
   
  

end
 
if init_reset == 0&& t>0
    reset = 1;
 
end

== matlab function ballonplate_correctordinates29062016/Coordinate_Transform_l_w1 ==
  data: x_vec input; y_vec input; x input; local output; y input; z input; world output
function [local,world]  = fcn(x_vec,y_vec,x,y,z)
%y_p is y prime which is vector of y coordinate axis after rotation beta
%about the x axis
%x_p is rotation alpha about arbitary axis y_p
%This transformation gives the coordinates in the mathematical model
%coordinates
%x_vec -1 0 0
%y_vec 0 0 1
%z_vec 0 1 0
% This gives local where x is -x therefore x is correct and z 
%just need to swap x and z
world = [x,y,z];
z_vec=cross(x_vec,y_vec);
local=[x_vec,y_vec,z_vec]\[x;y;z];


%this gives local coordinates in ball and plate frame
temp = local(1);
local(1) = local(2);
local(2) = temp;

== matlab function ballonplate_correctordinates29062016/Fall_off ==
  data: mod_sec input; mod_sec_edit output size=1; gravity data_store_memory; math_co input; bounce_co input; falloff_toggle data_store_memory; plate_dim_x input
function mod_sec_edit   = fcn(mod_sec,math_co,bounce_co,plate_dim_x)
%mod_sec if 0 output is bounce_co
%if anything else math_co
%this requires bounce_co and math_co for vrml model, note doesn't require
%the negative
%%%%29th june 2016 code
plate_dim_x = plate_dim_x/100;
%%%%%
% math_co;
plate_dim_y = plate_dim_x;
global gravity;
global falloff_toggle;


    if falloff_toggle ==0
        if mod_sec == 1;
            mod_sec_edit = 1;
            nates = bounce_co;
            if nates(2)<5&&(abs(nates(1)))>plate_dim_y||(abs(nates(3)))>plate_dim_y
                 mod_sec_edit = 3;
                 gravity = 0;
                 falloff_toggle = 1;
  
            end
        else mod_sec_edit = 0;
             nates = math_co;
                 if (abs(nates(1))) > plate_dim_x || (abs(nates(3))) > plate_dim_y
                    mod_sec_edit = 3; 
                    gravity = 0;
                    falloff_toggle = 1;
                 end
        end    
    else
        mod_sec_edit = 3;


    end
